simulink model "ramjet"  (R2019b)
settings: Solver=FixedStepAuto  StartTime=0.0  StopTime=10  FixedStep=0.3  RelTol=1e-3
undefined symbols (not defined in the file or in its folder): combustion, diffuser, inlet_v, nozzle
libraries: simulink_extras x1
settings Model: Creator=Administrator  LastModifiedBy=AJH
settings DataIOCC: ExternalInput=m_dot

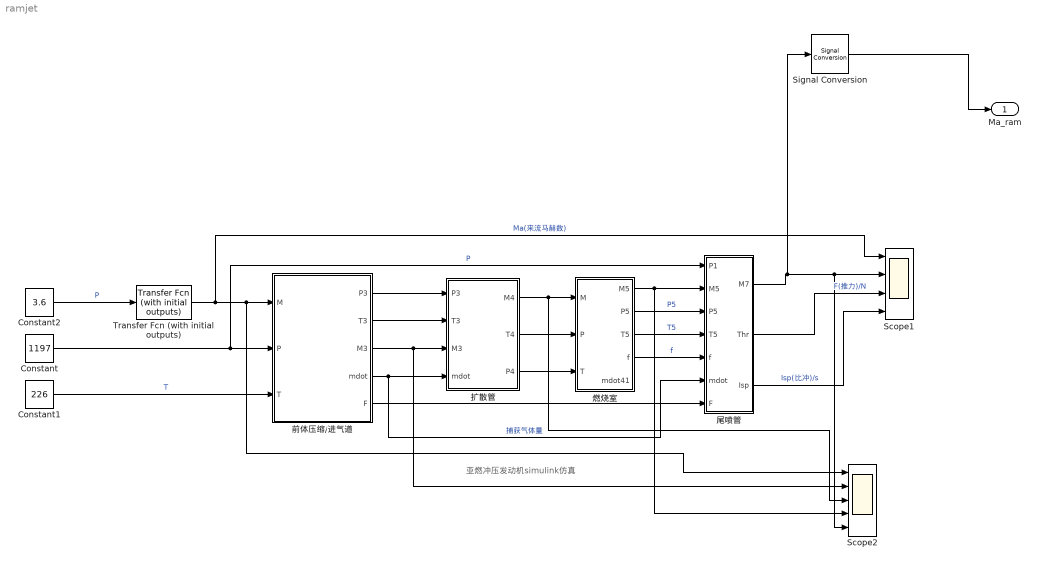
== system ramjet ==
  note: 亚燃冲压发动机simulink仿真
  Constant : Constant  Value=1197
  Constant1 : Constant  Value=226
  Constant2 : Constant  Value=3.6
  Scope1 : Scope  NumInputPorts=4
  Scope2 : Scope  NumInputPorts=5
  Signal Conversion : SignalConversion  OverrideOpt=off
  Transfer Fcn (with initial outputs) : simulink_extras/Additional Linear/Transfer Fcn (with initial outputs)  N=[1]  D="[2  1]"  Y0=2.6  U0=0
  前体压缩/进气道 : Subsystem
  尾喷管 : Subsystem
  扩散管 : Subsystem
  燃烧室 : Subsystem
  Ma_ram : Outport
  wires:
  Transfer Fcn (with initial outputs)/1 -> Scope1/1, Scope2/1, 前体压缩/进气道/1(M)  "Ma(来流马赫数)"
  Constant/1 -> 尾喷管/1(P1), 前体压缩/进气道/2(P)  "P"
  Constant1/1 -> 前体压缩/进气道/3(T)  "T"
  前体压缩/进气道/1(P3) -> 扩散管/1(P3)
  前体压缩/进气道/2(T3) -> 扩散管/2(T3)
  前体压缩/进气道/3(M3) -> Scope2/2, 扩散管/3(M3)
  前体压缩/进气道/4(mdot) -> 尾喷管/6(mdot), 扩散管/4(mdot)  "捕获气体量"
  扩散管/1(M4) -> Scope2/3, 燃烧室/1(M)
  扩散管/2(T4) -> 燃烧室/2(P)
  扩散管/3(P4) -> 燃烧室/3(T)
  燃烧室/1(M5) -> Scope2/4, 尾喷管/2(M5)
  燃烧室/2(P5) -> 尾喷管/3(P5)  "P5"
  燃烧室/3(T5) -> 尾喷管/4(T5)  "T5"
  燃烧室/4(f) -> 尾喷管/5(f)  "f"
  前体压缩/进气道/5(F) -> 尾喷管/7(F)
  尾喷管/2(Thr) -> Scope1/3  "F(推力)/N"
  尾喷管/3(Isp) -> Scope1/4  "Isp(比冲)/s"
  Constant2/1 -> Transfer Fcn (with initial outputs)/1  "P"
  Signal Conversion/1 -> Ma_ram/1
  尾喷管/1(M7) -> Signal Conversion/1, Scope1/2, Scope2/5

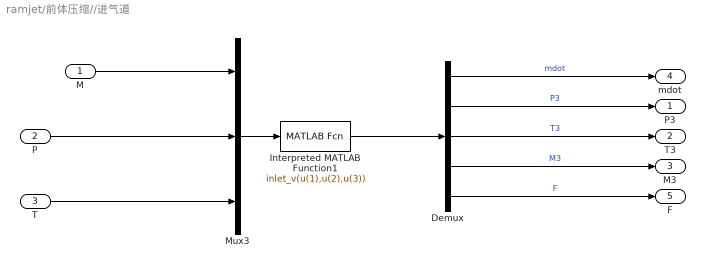
== system ramjet/前体压缩//进气道 ==
  M : Inport
  P : Inport  Port=2
  T : Inport  Port=3
  Demux : Demux  Outputs=5
  Interpreted MATLAB Function1 : MATLABFcn  MATLABFcn=inlet_v(u(1),u(2),u(3))  OutputDimensions=5
  Mux3 : Mux  Inputs=3
  P3 : Outport
  T3 : Outport  Port=2
  M3 : Outport  Port=3
  mdot : Outport  Port=4
  F : Outport  Port=5
  wires:
  Mux3/1 -> Interpreted MATLAB Function1/1
  Demux/1 -> mdot/1  "mdot"
  Interpreted MATLAB Function1/1 -> Demux/1
  M/1 -> Mux3/1
  P/1 -> Mux3/2
  Demux/5 -> F/1  "F"
  T/1 -> Mux3/3
  Demux/2 -> P3/1  "P3"
  Demux/3 -> T3/1  "T3"
  Demux/4 -> M3/1  "M3"

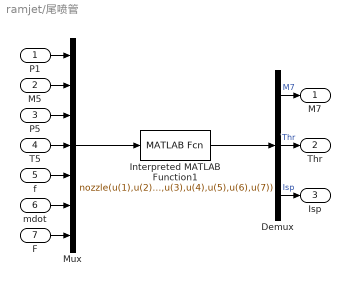
== system ramjet/尾喷管 ==
  P1 : Inport
  M5 : Inport  Port=2
  P5 : Inport  Port=3
  T5 : Inport  Port=4
  f : Inport  Port=5
  mdot : Inport  Port=6
  F : Inport  Port=7
  Demux : Demux  Outputs=3
  Interpreted MATLAB Function1 : MATLABFcn  MATLABFcn=nozzle(u(1),u(2),u(3),u(4),u(5),u(6),u(7))  OutputDimensions=3
  Mux : Mux  Inputs=7
  M7 : Outport
  Thr : Outport  Port=2
  Isp : Outport  Port=3
  wires:
  Demux/3 -> Isp/1  "Isp"
  f/1 -> Mux/5
  mdot/1 -> Mux/6
  Interpreted MATLAB Function1/1 -> Demux/1
  Mux/1 -> Interpreted MATLAB Function1/1
  P5/1 -> Mux/3
  Demux/1 -> M7/1  "M7"
  F/1 -> Mux/7
  Demux/2 -> Thr/1  "Thr"
  M5/1 -> Mux/2
  P1/1 -> Mux/1
  T5/1 -> Mux/4

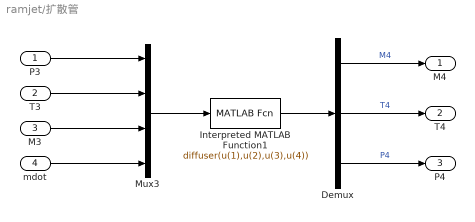
== system ramjet/扩散管 ==
  P3 : Inport
  T3 : Inport  Port=2
  M3 : Inport  Port=3
  mdot : Inport  Port=4
  Demux : Demux  Outputs=3
  Interpreted MATLAB Function1 : MATLABFcn  MATLABFcn=diffuser(u(1),u(2),u(3),u(4))  OutputDimensions=3
  Mux3 : Mux
  M4 : Outport
  T4 : Outport  Port=2
  P4 : Outport  Port=3
  wires:
  Demux/3 -> P4/1  "P4"
  T3/1 -> Mux3/2
  M3/1 -> Mux3/3
  Demux/2 -> T4/1  "T4"
  Interpreted MATLAB Function1/1 -> Demux/1
  Mux3/1 -> Interpreted MATLAB Function1/1
  mdot/1 -> Mux3/4
  P3/1 -> Mux3/1
  Demux/1 -> M4/1  "M4"

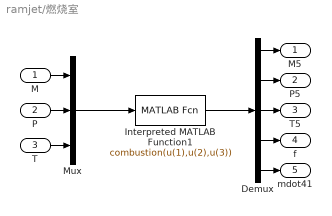
== system ramjet/燃烧室 ==
  M : Inport
  P : Inport  Port=2
  T : Inport  Port=3
  Demux : Demux  Outputs=5
  Interpreted MATLAB Function1 : MATLABFcn  MATLABFcn=combustion(u(1),u(2),u(3))  OutputDimensions=5
  Mux : Mux  Inputs=3
  M5 : Outport
  P5 : Outport  Port=2
  T5 : Outport  Port=3
  f : Outport  Port=4
  mdot41 : Outport  Port=5
  wires:
  Mux/1 -> Interpreted MATLAB Function1/1
  Demux/4 -> f/1
  M/1 -> Mux/1
  P/1 -> Mux/2
  Demux/3 -> T5/1
  Interpreted MATLAB Function1/1 -> Demux/1
  Demux/5 -> mdot41/1
  Demux/2 -> P5/1
  Demux/1 -> M5/1
  T/1 -> Mux/3
